simulink model "CAN_T"  (R2018a)
settings: Solver=VariableStepAuto  StartTime=0.0  StopTime=10  RelTol=1e-3
undefined symbols (not defined in the file): A_Temp, canChannel, RPM, Throttle, W_Temp
libraries: simulink x10, canlib x2, canmsglib x1
settings Model: Creator=arthu  LastModifiedBy=arthu

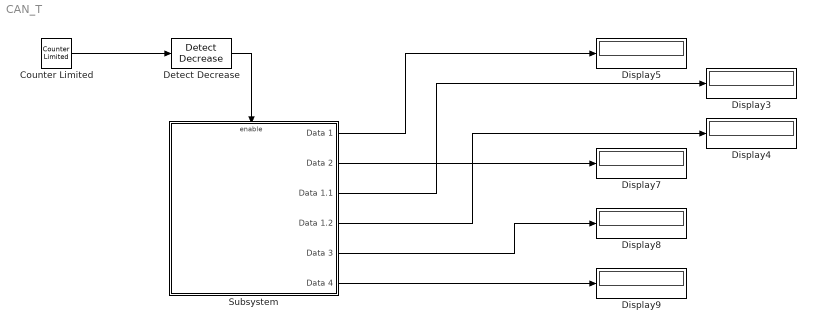
== system CAN_T ==
  Counter Limited : simulink/Sources/Counter Limited  uplimit=24  tsamp=0.001
  Detect Decrease : simulink/Logic and Bit Operations/Detect Decrease  vinit=0.0  OutDataTypeStr=boolean
  Display{3..5,7..9} (6 alike) : Display
  Subsystem : Subsystem
  wires:
  Detect Decrease/1 -> Subsystem/Enable
  Counter Limited/1 -> Detect Decrease/1
  Subsystem/3(Data 1.1) -> Display3/1
  Subsystem/4(Data 1.2) -> Display4/1
  Subsystem/1(Data 1) -> Display5/1
  Subsystem/2(Data 2) -> Display7/1
  Subsystem/6(Data 4) -> Display9/1
  Subsystem/5("Data 3 ") -> Display8/1

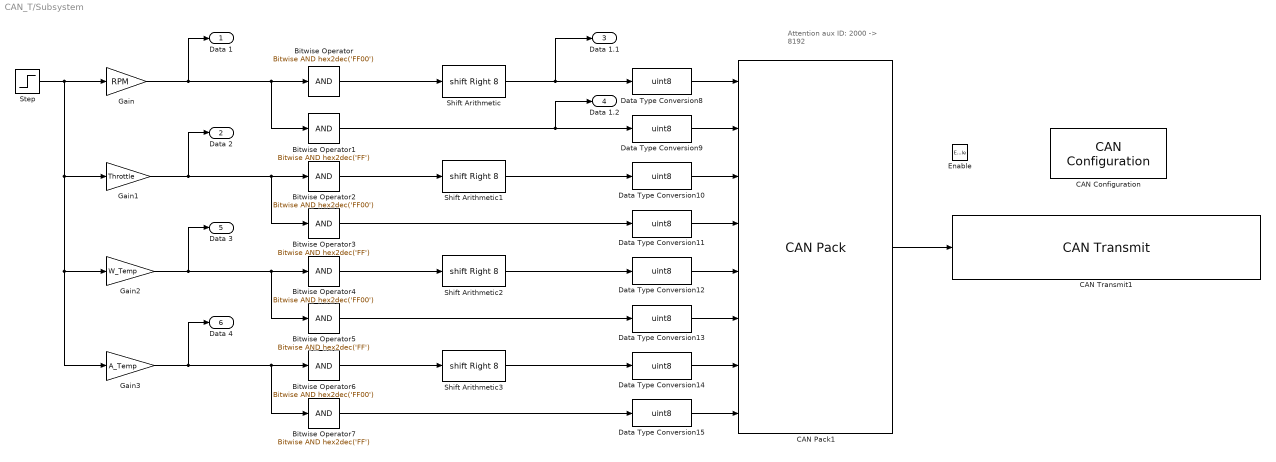
== system CAN_T/Subsystem ==
  note: Attention aux ID:
      | 2000 -> 8192
  Enable : EnablePort
  Bitwise Operator{,2,4,6} (4 alike) : simulink/Logic and Bit Operations/Bitwise Operator  logicop=AND  UseBitMask=on  BitMask=hex2dec('FF00')  BitMaskRealWorld=Stored Integer
  Bitwise Operator{1,3,5,7} (4 alike) : simulink/Logic and Bit Operations/Bitwise Operator  logicop=AND  UseBitMask=on  BitMask=hex2dec('FF')  BitMaskRealWorld=Stored Integer
  CAN Configuration : canlib/CAN Configuration  BlockHandle=33.0002  DeviceMenu=MathWorks Virtual 1 (Channel 1)  Device=PEAK-System PCAN-USB (PCAN_USBBUS1)  ObjConstructor=canChannel('PEAK-System','PCAN_USBBUS1')  BusSpeed=1000000  EnableBitParameters=off  AckMode=Normal
      settings: SourceProductName=Vehicle Network Toolbox  SourceProductBaseCode=VN
  CAN Pack1 : canmsglib/CAN Pack  MsgList=(none)  MsgName=CAN Msg  MsgIDType=Extended (29-bit identifier)  MsgIdentifier=8192  MsgLength=8  SignalInfo=Signal1$0$8$1$2$1$0$1$0$-Inf$Inf$#Signal2$8$8$1$2$1$0$1$0$-Inf$Inf$#Signal3$16$8$1$2$1$0$1$0$-Inf$Inf$#Signal4$24$8$1$2$1$0$1$0$-Inf$Inf$#Signal5$32$8$1$2$1$0$1$0$-Inf$Inf$#Signal6$40$8$1$2$1$0$1$0$-Inf$Inf$#Signal7$48$8$1$2$1$0$1$0$-Inf$Inf$#Signal8$56$8$1$2$1$0$1$0$-Inf$Inf$#  NSignals=8  StartBits=str2num('[int32(0);int32(8);int32(16);int32(24);int32(32);int32(40);int32(48);int32(56)]')  SignalSizes=str2num('[int32(8);int32(8);int32(8);int32(8);int32(8);int32(8);int32(8);int32(8)]')  ByteOrders=str2num('[int32(1);int32(1);int32(1);int32(1);int32(1);int32(1);int32(1);int32(1)]')  DataTypes=str2num('[int32(2);int32(2);int32(2);int32(2);int32(2);int32(2);int32(2);int32(2)]')  MultiplexTypes=str2num('[int32(1);int32(1);int32(1);int32(1);int32(1);int32(1);int32(1);int32(1)]')  MultiplexValues=str2num('[double(0);double(0);double(0);double(0);double(0);double(0);double(0);double(0)]')  Factors=str2num('[double(1);double(1);double(1);double(1);double(1);double(1);double(1);double(1)]')  Offsets=str2num('[double(0);double(0);double(0);double(0);double(0);double(0);double(0);double(0)]')  Minimums=str2num('[double(-Inf);double(-Inf);double(-Inf);double(-Inf);double(-Inf);double(-Inf);double(-Inf);double(-Inf)]')  Maximums=str2num('[double(Inf);double(Inf);double(Inf);double(Inf);double(Inf);double(Inf);double(Inf);double(Inf)]')  Remote=off  ApplyMinMax=off  BusOutput=off
      settings: SourceProductName=Simulink Real-Time  SourceProductBaseCode=XP  DataFormat=manually specified signals
  CAN Transmit1 : canlib/CAN Transmit  BlockHandle=37.0002  DeviceMenu=MathWorks Virtual 1 (Channel 1)  Device=PEAK-System PCAN-USB (PCAN_USBBUS1)  ObjConstructor=canChannel('PEAK-System','PCAN_USBBUS1')  EnablePeriodicTransmit=off  MessagePeriod=0.050
      settings: SourceProductName=Vehicle Network Toolbox  SourceProductBaseCode=VN
  Data Type Conversion{8..15} (8 alike) : DataTypeConversion  OutDataTypeStr=uint8
  Gain : Gain  Gain=RPM  OutDataTypeStr=uint16
  Gain1 : Gain  Gain=Throttle  OutDataTypeStr=uint16
  Gain2 : Gain  Gain=W_Temp  OutDataTypeStr=uint16
  Gain3 : Gain  Gain=A_Temp  OutDataTypeStr=uint16
  Shift Arithmetic{,1..3} (4 alike) : ArithShift  BitShiftNumber=8  BitShiftDirection=Right
  Step : Step  Time=0
  Data 1 : Outport
  Data 2 : Outport  Port=2
  Data 1.1 : Outport  Port=3
  Data 1.2 : Outport  Port=4
  "Data 3 " : Outport  Port=5
  Data 4 : Outport  Port=6
  wires:
  CAN Pack1/1 -> CAN Transmit1/1
  Data Type Conversion8/1 -> CAN Pack1/1
  Data Type Conversion9/1 -> CAN Pack1/2
  Data Type Conversion10/1 -> CAN Pack1/3
  Data Type Conversion11/1 -> CAN Pack1/4
  Data Type Conversion12/1 -> CAN Pack1/5
  Data Type Conversion13/1 -> CAN Pack1/6
  Data Type Conversion14/1 -> CAN Pack1/7
  Data Type Conversion15/1 -> CAN Pack1/8
  Bitwise Operator/1 -> Shift Arithmetic/1
  Bitwise Operator1/1 -> Data 1.2/1, Data Type Conversion9/1
  Shift Arithmetic/1 -> Data 1.1/1, Data Type Conversion8/1
  Bitwise Operator3/1 -> Data Type Conversion11/1
  Bitwise Operator2/1 -> Shift Arithmetic1/1
  Shift Arithmetic1/1 -> Data Type Conversion10/1
  Bitwise Operator4/1 -> Shift Arithmetic2/1
  Bitwise Operator5/1 -> Data Type Conversion13/1
  Shift Arithmetic2/1 -> Data Type Conversion12/1
  Bitwise Operator7/1 -> Data Type Conversion15/1
  Bitwise Operator6/1 -> Shift Arithmetic3/1
  Shift Arithmetic3/1 -> Data Type Conversion14/1
  Gain/1 -> Data 1/1, Bitwise Operator1/1, Bitwise Operator/1
  Gain1/1 -> Bitwise Operator3/1, Bitwise Operator2/1, Data 2/1
  Gain2/1 -> "Data 3 "/1, Bitwise Operator5/1, Bitwise Operator4/1
  Gain3/1 -> Data 4/1, Bitwise Operator7/1, Bitwise Operator6/1
  Step/1 -> Gain2/1, Gain3/1, Gain1/1, Gain/1
